simulink model "estimator_ekf_v04"  (Simulink 7.0)
settings: Solver=FixedStepDiscrete  StartTime=10  StopTime=20  FixedStep=1e-3  RelTol=1e-3
undefined symbols (not defined in the file): Ilf, Irf, P0, Q_in, R, ROBOT, ts, X0
libraries: simulink x6
settings Model: Creator=raje_ra  LastModifiedBy=raje_ra  ExtModeAutoUpdateStatusClock=off
settings DebuggingCC: SignalInfNanChecking=error  CheckMatrixSingularityMsg=warning

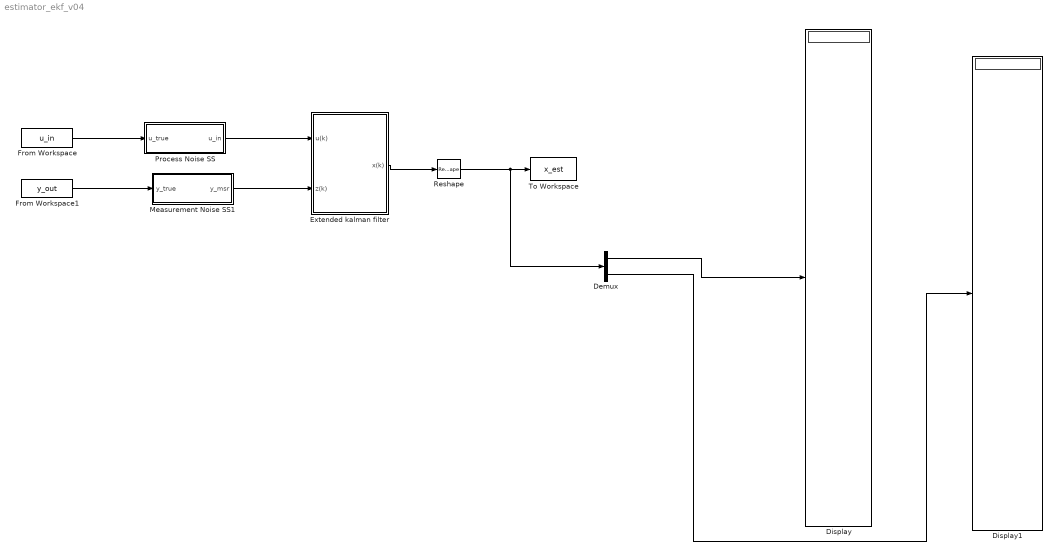
== system estimator_ekf_v04 ==
  Demux : Demux  Outputs=2
  Display : Display
  Display1 : Display
  Extended kalman filter : Subsystem
  From Workspace : FromWorkspace  VariableName=u_in  SampleTime=0
  From Workspace1 : FromWorkspace  VariableName=y_out  SampleTime=0
  Measurement Noise SS1 : Subsystem
  Process Noise SS : Subsystem
  Reshape : Reshape
  To Workspace : ToWorkspace  VariableName=x_est  SampleTime=-1  SaveFormat=Structure With Time
  wires:
  Extended kalman filter/1(x(k)) -> Reshape/1
  From Workspace1/1 -> Measurement Noise SS1/1(y_true)
  From Workspace/1 -> Process Noise SS/1(u_true)
  Reshape/1 -> To Workspace/1, Demux/1
  Measurement Noise SS1/1(y_msr) -> Extended kalman filter/2(z(k))
  Demux/1 -> Display/1
  Demux/2 -> Display1/1
  Process Noise SS/1(u_in) -> Extended kalman filter/1(u(k))

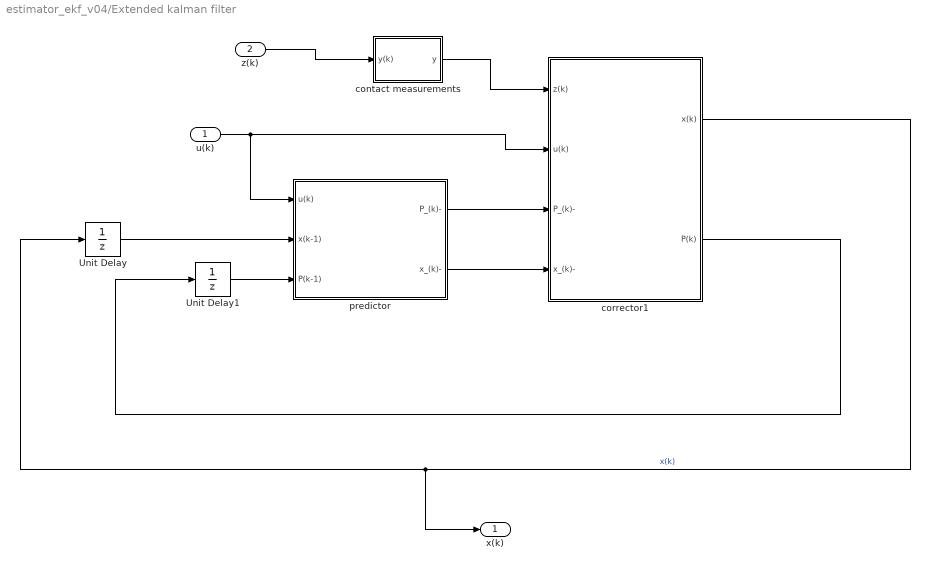
== system estimator_ekf_v04/Extended kalman filter ==
  u(k) : Inport  OutDataType=sfix(16)  OutScaling=2^0
  z(k) : Inport  Port=2  OutDataType=sfix(16)  OutScaling=2^0
  Unit Delay : UnitDelay  X0=X0  SampleTime=ts
  Unit Delay1 : UnitDelay  X0=P0  SampleTime=ts
  contact measurements : Subsystem
  corrector1 : Subsystem
  predictor : Subsystem
  x(k) : Outport  OutDataType=sfix(16)  OutScaling=2^0
  wires:
  u(k)/1 -> predictor/1(u(k)), corrector1/2(u(k))
  predictor/2(x_(k)-) -> corrector1/4(x_(k)-)
  Unit Delay/1 -> predictor/2(x(k-1))
  Unit Delay1/1 -> predictor/3(P(k-1))
  predictor/1(P_(k)-) -> corrector1/3(P_(k)-)
  corrector1/1(x(k)) -> Unit Delay/1, x(k)/1  "x(k)"
  z(k)/1 -> contact measurements/1(y(k))
  contact measurements/1(y) -> corrector1/1(z(k))
  corrector1/2(P(k)) -> Unit Delay1/1

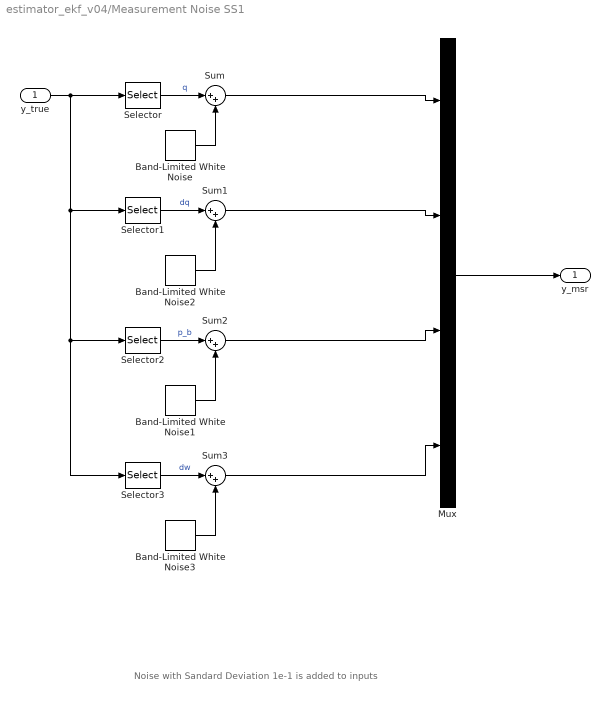
== system estimator_ekf_v04/Measurement Noise SS1 ==
  note: Noise with Sandard Deviation 1e-1 is added to inputs
  y_true : Inport  OutDataType=sfix(16)  OutScaling=2^0
  Band-Limited White Noise : simulink/Sources/Band-Limited White Noise  SystemSampleTime=-1  Cov=[1e-9]  Ts=ts  seed=[23341]
  Band-Limited White Noise1 : simulink/Sources/Band-Limited White Noise  SystemSampleTime=-1  Cov=[1e-5]  Ts=ts  seed=[23341]
  Band-Limited White Noise2 : simulink/Sources/Band-Limited White Noise  SystemSampleTime=-1  Cov=[1e-7]  Ts=ts  seed=[23341]
  Band-Limited White Noise3 : simulink/Sources/Band-Limited White Noise  SystemSampleTime=-1  Cov=[1e-7]  Ts=ts  seed=[23341]
  Mux : Mux
  Selector : Selector  InputPortWidth=m  IndexOptions=Index vector (dialog)  Indices=[1:25]  OutputSizes=1
  Selector1 : Selector  InputPortWidth=m  IndexOptions=Index vector (dialog)  Indices=[26:50]  OutputSizes=1
  Selector2 : Selector  InputPortWidth=m  IndexOptions=Index vector (dialog)  Indices=[51:53]  OutputSizes=1
  Selector3 : Selector  InputPortWidth=m  IndexOptions=Index vector (dialog)  Indices=[54:56]  OutputSizes=1
  Sum{,1..3} (4 alike) : Sum  Inputs=|++  OutDataType=sfix(16)  OutScaling=2^0
  y_msr : Outport
  wires:
  Mux/1 -> y_msr/1
  Sum3/1 -> Mux/4
  Sum2/1 -> Mux/3
  Sum1/1 -> Mux/2
  Sum/1 -> Mux/1
  Selector3/1 -> Sum3/1  "dw"
  Band-Limited White Noise3/1 -> Sum3/2
  Selector2/1 -> Sum2/1  "p_b"
  Band-Limited White Noise1/1 -> Sum2/2
  Band-Limited White Noise2/1 -> Sum1/2
  Selector1/1 -> Sum1/1  "dq"
  Selector/1 -> Sum/1  "q"
  y_true/1 -> Selector3/1, Selector2/1, Selector1/1, Selector/1
  Band-Limited White Noise/1 -> Sum/2

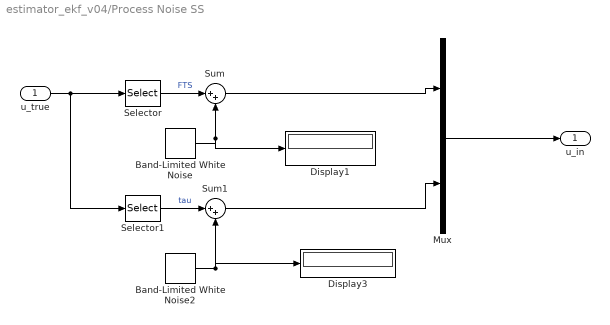
== system estimator_ekf_v04/Process Noise SS ==
  u_true : Inport  OutDataType=sfix(16)  OutScaling=2^0
  Band-Limited White Noise : simulink/Sources/Band-Limited White Noise  SystemSampleTime=-1  Cov=[1e-5]  Ts=ts  seed=[23341]
  Band-Limited White Noise2 : simulink/Sources/Band-Limited White Noise  SystemSampleTime=-1  Cov=[1e-6]  Ts=ts  seed=[23341]
  Display1 : Display
  Display3 : Display
  Mux : Mux  Inputs=2
  Selector : Selector  InputPortWidth=37  IndexOptions=Index vector (dialog)  Indices=[1:12]  OutputSizes=1
  Selector1 : Selector  InputPortWidth=37  IndexOptions=Index vector (dialog)  Indices=[13:37]  OutputSizes=1
  Sum : Sum  Inputs=|++  OutDataType=sfix(16)  OutScaling=2^0
  Sum1 : Sum  Inputs=|++  OutDataType=sfix(16)  OutScaling=2^0
  u_in : Outport
  wires:
  Mux/1 -> u_in/1
  Sum1/1 -> Mux/2
  Sum/1 -> Mux/1
  Band-Limited White Noise2/1 -> Display3/1, Sum1/2
  Selector1/1 -> Sum1/1  "tau"
  Selector/1 -> Sum/1  "FTS"
  u_true/1 -> Selector/1, Selector1/1
  Band-Limited White Noise/1 -> Display1/1, Sum/2

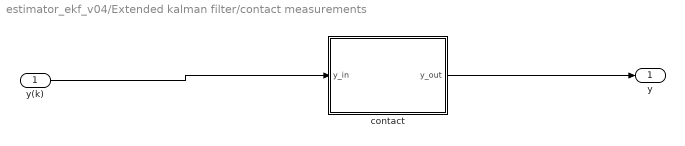
== system estimator_ekf_v04/Extended kalman filter/contact measurements ==
  y(k) : Inport
  contact : Subsystem  TreatAsAtomicUnit=on
  y : Outport
  wires:
  contact/1(y_out) -> y/1
  y(k)/1 -> contact/1(y_in)

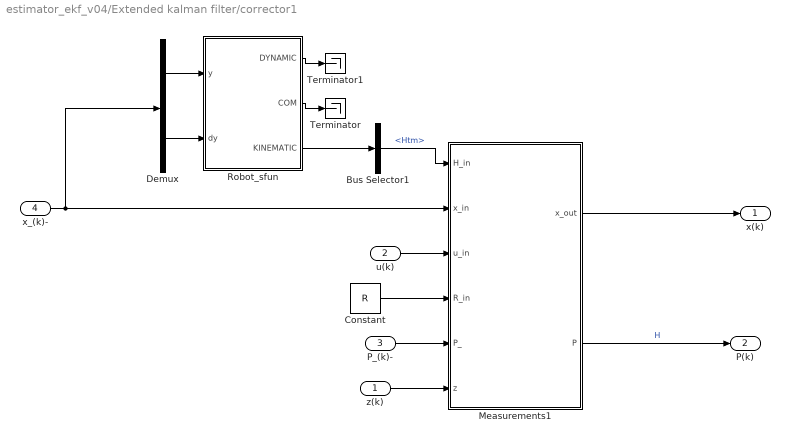
== system estimator_ekf_v04/Extended kalman filter/corrector1 ==
  z(k) : Inport  OutDataType=sfix(16)  OutScaling=2^0
  u(k) : Inport  Port=2  OutDataType=sfix(16)  OutScaling=2^0
  P_(k)- : Inport  Port=3  OutDataType=sfix(16)  OutScaling=2^0
  x_(k)- : Inport  Port=4  OutDataType=sfix(16)  OutScaling=2^0
  Bus Selector1 : BusSelector  OutputSignals=Htm
  Constant : Constant  Value=R  OutDataType=sfix(16)  OutScaling=2^0
  Demux : Demux  Outputs=2
  Measurements1 : Stateflow chart
  Robot_sfun : Subsystem
  Terminator : Terminator
  Terminator1 : Terminator
  x(k) : Outport  OutDataType=sfix(16)  OutScaling=2^0
  P(k) : Outport  Port=2  OutDataType=sfix(16)  OutScaling=2^0
  wires:
  Measurements1/2(P) -> P(k)/1  "H"
  z(k)/1 -> Measurements1/6(z)
  Constant/1 -> Measurements1/4(R_in)
  P_(k)-/1 -> Measurements1/5(P_)
  u(k)/1 -> Measurements1/3(u_in)
  Measurements1/1(x_out) -> x(k)/1
  x_(k)-/1 -> Measurements1/2(x_in), Demux/1
  Robot_sfun/2(COM) -> Terminator/1
  Demux/2 -> Robot_sfun/2(dy)
  Demux/1 -> Robot_sfun/1(y)
  Bus Selector1/1 -> Measurements1/1(H_in)  "<Htm>"
  Robot_sfun/3(KINEMATIC) -> Bus Selector1/1
  Robot_sfun/1(DYNAMIC) -> Terminator1/1

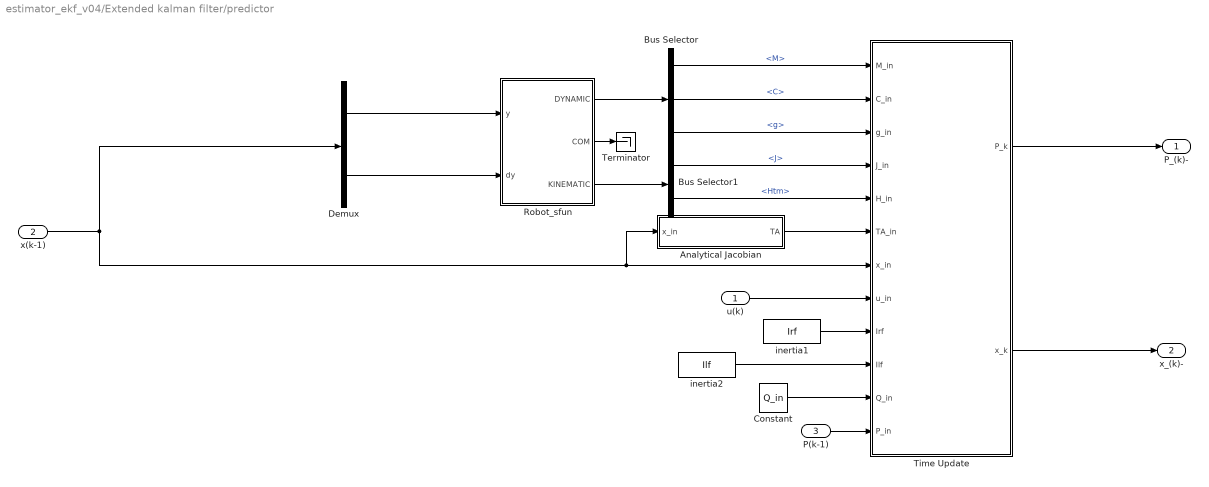
== system estimator_ekf_v04/Extended kalman filter/predictor ==
  u(k) : Inport  OutDataType=sfix(16)  OutScaling=2^0
  x(k-1) : Inport  Port=2  OutDataType=sfix(16)  OutScaling=2^0
  P(k-1) : Inport  Port=3  OutDataType=sfix(16)  OutScaling=2^0
  Analytical Jacobian : Stateflow chart
  Bus Selector : BusSelector  OutputSignals=M,C,g
  Bus Selector1 : BusSelector  OutputSignals=J,Htm
  Constant : Constant  Value=Q_in  VectorParams1D=off  OutDataType=sfix(16)  OutScaling=2^0
  Demux : Demux  Outputs=2
  Robot_sfun : Subsystem
  Terminator : Terminator
  Time Update : Stateflow chart
  inertia1 : Constant  Value=Irf  VectorParams1D=off  OutDataType=sfix(16)  OutScaling=2^0
  inertia2 : Constant  Value=Ilf  VectorParams1D=off  OutDataType=sfix(16)  OutScaling=2^0
  P_(k)- : Outport  OutDataType=sfix(16)  OutScaling=2^0
  x_(k)- : Outport  Port=2  OutDataType=sfix(16)  OutScaling=2^0
  wires:
  Time Update/1(P_k) -> P_(k)-/1
  Constant/1 -> Time Update/11(Q_in)
  P(k-1)/1 -> Time Update/12(P_in)
  Time Update/2(x_k) -> x_(k)-/1
  inertia2/1 -> Time Update/10(Ilf)
  inertia1/1 -> Time Update/9(Irf)
  u(k)/1 -> Time Update/8(u_in)
  Analytical Jacobian/1(TA) -> Time Update/6(TA_in)
  Robot_sfun/2(COM) -> Terminator/1
  Demux/2 -> Robot_sfun/2(dy)
  Demux/1 -> Robot_sfun/1(y)
  x(k-1)/1 -> Demux/1, Time Update/7(x_in), Analytical Jacobian/1(x_in)
  Bus Selector1/2 -> Time Update/5(H_in)  "<Htm>"
  Bus Selector1/1 -> Time Update/4(J_in)  "<J>"
  Robot_sfun/3(KINEMATIC) -> Bus Selector1/1
  Bus Selector/3 -> Time Update/3(g_in)  "<g>"
  Bus Selector/2 -> Time Update/2(C_in)  "<C>"
  Bus Selector/1 -> Time Update/1(M_in)  "<M>"
  Robot_sfun/1(DYNAMIC) -> Bus Selector/1

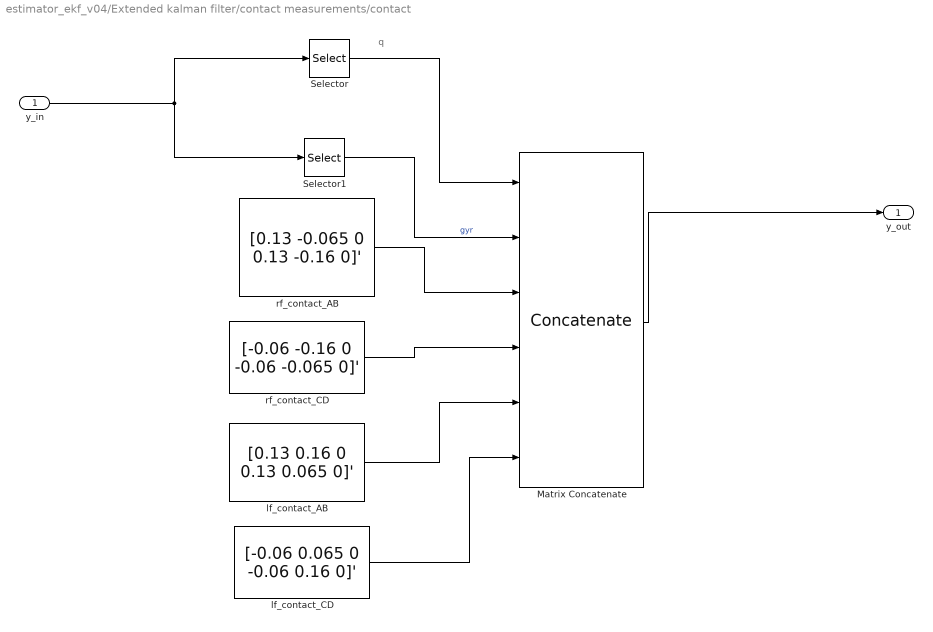
== system estimator_ekf_v04/Extended kalman filter/contact measurements/contact ==
  note: q
  y_in : Inport  OutDataType=sfix(16)  OutScaling=2^0
  Matrix Concatenate : Concatenate  NumInputs=6  Mode=Multidimensional array
  Selector : Selector  InputPortWidth=56  IndexOptions=Index vector (dialog)  Indices=1:25  OutputSizes=1
  Selector1 : Selector  InputPortWidth=56  IndexOptions=Index vector (dialog)  Indices=54:56  OutputSizes=1
  lf_contact_AB : Constant  Value="[0.13  0.16  0  0.13  0.065  0]'"  VectorParams1D=off  OutDataType=sfix(16)  OutScaling=2^0
  lf_contact_CD : Constant  Value="[-0.06  0.065  0  -0.06  0.16 0]'"  VectorParams1D=off  OutDataType=sfix(16)  OutScaling=2^0
  rf_contact_AB : Constant  Value="[0.13  -0.065  0   0.13  -0.16  0]'"  VectorParams1D=off  OutDataType=sfix(16)  OutScaling=2^0
  rf_contact_CD : Constant  Value="[-0.06  -0.16  0  -0.06  -0.065 0]'"  VectorParams1D=off  OutDataType=sfix(16)  OutScaling=2^0
  y_out : Outport  OutDataType=sfix(16)  OutScaling=2^0
  wires:
  lf_contact_CD/1 -> Matrix Concatenate/6
  lf_contact_AB/1 -> Matrix Concatenate/5
  rf_contact_CD/1 -> Matrix Concatenate/4
  rf_contact_AB/1 -> Matrix Concatenate/3
  Selector1/1 -> Matrix Concatenate/2  "gyr"
  Selector/1 -> Matrix Concatenate/1
  y_in/1 -> Selector1/1, Selector/1
  Matrix Concatenate/1 -> y_out/1

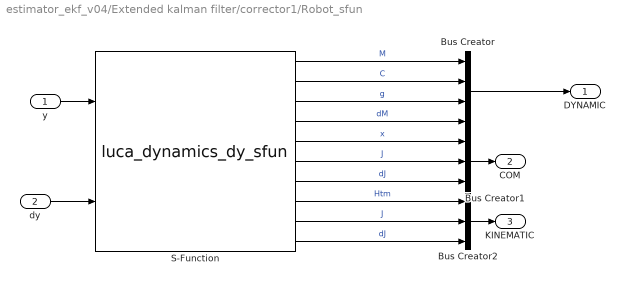
== system estimator_ekf_v04/Extended kalman filter/corrector1/Robot_sfun ==
  y : Inport
  dy : Inport  Port=2
  Bus Creator : BusCreator
  Bus Creator1 : BusCreator  Inputs=3
  Bus Creator2 : BusCreator  Inputs=3
  S-Function : S-Function  FunctionName=luca_dynamics_dy_sfun  Parameters=(size(ROBOT.csi,1)/6-1), size(ROBOT.csi,2), ROBOT.parent, ROBOT.tcp, ROBOT.g0, ROBOT.csi, ROBOT.com, ROBOT.Mass
  DYNAMIC : Outport
  COM : Outport  Port=2
  KINEMATIC : Outport  Port=3
  wires:
  Bus Creator2/1 -> KINEMATIC/1
  Bus Creator1/1 -> COM/1
  Bus Creator/1 -> DYNAMIC/1
  S-Function/10 -> Bus Creator2/3  "dJ"
  S-Function/9 -> Bus Creator2/2  "J"
  S-Function/8 -> Bus Creator2/1  "Htm"
  S-Function/7 -> Bus Creator1/3  "dJ"
  S-Function/6 -> Bus Creator1/2  "J"
  S-Function/5 -> Bus Creator1/1  "x"
  S-Function/4 -> Bus Creator/4  "dM"
  S-Function/3 -> Bus Creator/3  "g"
  S-Function/2 -> Bus Creator/2  "C"
  S-Function/1 -> Bus Creator/1  "M"
  dy/1 -> S-Function/2
  y/1 -> S-Function/1

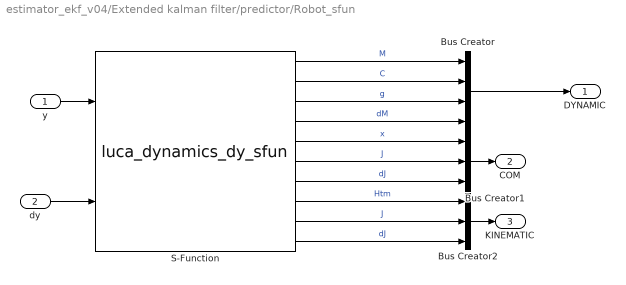
== system estimator_ekf_v04/Extended kalman filter/predictor/Robot_sfun ==
  y : Inport
  dy : Inport  Port=2
  Bus Creator : BusCreator
  Bus Creator1 : BusCreator  Inputs=3
  Bus Creator2 : BusCreator  Inputs=3
  S-Function : S-Function  FunctionName=luca_dynamics_dy_sfun  Parameters=(size(ROBOT.csi,1)/6-1), size(ROBOT.csi,2), ROBOT.parent, ROBOT.tcp, ROBOT.g0, ROBOT.csi, ROBOT.com, ROBOT.Mass
  DYNAMIC : Outport
  COM : Outport  Port=2
  KINEMATIC : Outport  Port=3
  wires:
  y/1 -> S-Function/1
  dy/1 -> S-Function/2
  S-Function/1 -> Bus Creator/1  "M"
  S-Function/2 -> Bus Creator/2  "C"
  S-Function/3 -> Bus Creator/3  "g"
  S-Function/4 -> Bus Creator/4  "dM"
  S-Function/5 -> Bus Creator1/1  "x"
  S-Function/6 -> Bus Creator1/2  "J"
  S-Function/7 -> Bus Creator1/3  "dJ"
  S-Function/8 -> Bus Creator2/1  "Htm"
  S-Function/9 -> Bus Creator2/2  "J"
  S-Function/10 -> Bus Creator2/3  "dJ"
  Bus Creator/1 -> DYNAMIC/1
  Bus Creator1/1 -> COM/1
  Bus Creator2/1 -> KINEMATIC/1

== matlab function Extended kalman filter/predictor/Analytical Jacobian ==
  data: TA output inherited; x_in input inherited
function TA = fcn(x_in)
% This block supports the Embedded MATLAB subset.
% See the help menu for details. 
% state - [ position ; velocity ]
% x_in  - [   1:31   ;   32:62  ]
ox = x_in(4);
oy = x_in(5);
% Transformation for Angular velocities to angular rates of floating base 
% on instantaneous frame of reference. x-y-z rotations.
%%{
T = [1      0           sin(oy);...
     0 cos(ox) -cos(oy)*sin(ox);...
     0 sin(ox)  cos(oy)*cos(ox)];


dTx = [0,         0,                0 ;...
       0,  -sin(ox),  -cos(oy)*cos(ox);...
       0,   cos(ox),  -cos(oy)*sin(ox)];
dTy = [0,         0,           cos(oy);...
       0,         0,   sin(oy)*sin(ox);...
       0,         0,  -sin(oy)*cos(ox)];
%%}

%{
T = [1      0   -sin(oy);...
     0  cos(ox)  cos(oy)*sin(ox);...
     0 -sin(ox)  cos(oy)*cos(ox)];
 
%T_A = [eye(3,6);zeros(3),T];

dTx = [0         0                0 ;
       0   -sin(ox)  cos(oy)*cos(ox);
       0   -cos(ox) -cos(oy)*sin(ox)];
dTy = [0       0        -cos(oy);
       0       0        -sin(oy)*sin(ox);
       0       0        -sin(oy)*cos(ox)];
%}

%TA = [ T_A; zeros(3*6,6); [zeros(3,6); [zeros(3) dTx]] ; [zeros(3,6); [zeros(3) dTy]]; zeros(57*6,6) ];

TA = [ T; dTx;dTy;zeros(3,3)];

== matlab function Extended kalman filter/predictor/Time Update ==
  data: P_k output inherited; M_in input inherited; x_k output inherited; C_in input inherited; g_in input inherited; J_in input inherited; H_in input inherited; TA_in input inherited; x_in input inherited; u_in input inherited; Irf input inherited; Ilf input inherited; Q_in input inherited; P_in input inherited
function [P_k,x_k]= fcn(M_in,C_in,g_in,J_in,H_in,TA_in,x_in,u_in,Irf,Ilf,Q_in,P_in)
% This block supports the Embedded MATLAB subset.
% See the help menu for details. 

dt = 1e-3;
dof = 31;
ind4 = -3:0;
ind6 = -5:0;

% Dynamic parameters
M = M_in(1:dof,:);
C = C_in(1:dof,:);
grav = g_in(1:dof);

invM = M \ eye(dof,dof);
% Kinematics
% tcp = 1 - Right Foot ; 2 - Left Foot ; 3 - Right Hand ; 4 - Left Hand ;
%       5 - Floating Base

Jrf = J_in(1*6+ind6,:);
Jlf = J_in(2*6+ind6,:);

Hrf = H_in(1*4+ind4,:);
Rrf = Hrf(1:3,1:3);
prf = Skew(Hrf(1:3,4));

Hlf = H_in(2*4+ind4,:);
Rlf = Hlf(1:3,1:3);
plf = Skew(Hlf(1:3,4));

Hfb = H_in(5*4+ind4,:);
Rfb = Hfb(1:3,1:3);

% state - [ position ; velocity ]
% x_in  - [   1:31   ;   32:62  ]
%q = x_in(1:dof);
dq = x_in(dof+(1:dof));

% inputs - [FTS_RF ; FTS _LF ; TRQ_JOINT]
% u_in   - [  1:6  ;   7:12  ;  13:37   ]
Frf = u_in(1*6+ind6,:);
Flf = u_in(2*6+ind6,:);
tau = [zeros(6,1); u_in(13:37)];

% Transformation for Angular velocities to angular rates of floating base 
% on instantaneous frame of reference. x-y-z rotations.
TA = TA_in(1:3,:);
invTA = TA \ eye(3,3);
% Transformation from body to spacial frame:
%Adfb = Adjoint(Hfb);
Adrf = Adjoint(Hrf);
Adlf = Adjoint(Hlf);

invAdrf = InvAdjoint(Hrf);
invAdlf = InvAdjoint(Hlf);

% Transformation for the velocites of floating base
vfb = dq(1:3);
wfb = dq(4:6);

dp = Rfb * vfb;
do = invTA * (Rfb*wfb);

vel = [dp; do; dq(7:31)];

%vel = [Vfb_s; dq(7:31)];%~~~~~~~ First Attempt

gacc = [ 0 0 -9.81 0 0 0]';
errrf = Irf * invAdrf * gacc ;
errlf = Ilf * invAdlf * gacc ;


% Computation of accelerations
acc = invM * (-C*dq - grav + tau + Jrf'*Adrf'*Frf + Jlf'*Adlf'*Flf - Jrf'*errrf - Jlf'*errlf);
x_dot = [vel;acc];   

% Computing second order derivative terms for base
% p - position of floating base o-orientation of floating base
x_k = x_in + dt*x_dot ;

% Computation the Jacobian of joint velocity function
dqdx = [zeros(25,37),eye(25)];                               %%%%%%%%%%%%%%%%

% Compute the Jacobian of acceleration terms(forward dynamics):
dpdx = zeros(3,2*dof);
dodx = zeros(3,2*dof);
dacc = zeros(dof,2*dof);
for i = 1:62
    dM   = M_in(i*dof+(1:dof),:);
    dC   = C_in(i*dof+(1:dof),:);
    dg   = g_in(i*dof+(1:dof));
    dJrf = J_in(i*30+(1*6+ind6),:);
    dJlf = J_in(i*30+(2*6+ind6),:);
    
    dHrf = H_in(i*20+(1*4+ind4),:);
    dRrf = dHrf(1:3,1:3);
    dprf = Skew(dHrf(1:3,4));
    dAdrf   = [ dRrf dprf*Rrf+prf*dRrf ; zeros(3) dRrf ];
    
    dHlf = H_in(i*20+(2*4+ind4),:); 
    dRlf = dHlf(1:3,1:3);
    dplf = Skew(dHlf(1:3,4));
    dAdlf   = [ dRlf dplf*Rlf+plf*dRlf ; zeros(3) dRlf ];
    
    dHfb  = H_in(i*20+(5*4+ind4),:); 
    dRfb  = dHfb( 1:3, 1:3);
 
    dpdx(:,i) = dRfb*vfb;
    dodx(:,i) = invTA * ( dRfb*wfb) ;

    if i > 3 && i < 6      
        dTA   = TA_in((i-3)*3+(1:3),:);
        dodx(:,i) = dodx(:,i) - invTA *(dTA*do );     % do = invTA * (Rfb*wfb);
    end 

      dacc(:,i)   = invM * (-dM*acc +(-dC*dq - dg + dJrf'*Adrf'*Frf + Jrf'*dAdrf'*Frf...
                                              + dJlf'*Adlf'*Flf + Jlf'*dAdlf'*Flf...
                                              - ( dJrf'*Irf* (invAdrf * gacc) + Jrf'*(-invAdrf *(dAdrf*(invAdrf * gacc))) ) ...
                                              - ( dJlf'*Ilf* (invAdlf * gacc) + Jlf'*(-invAdlf *(dAdlf*(invAdlf * gacc))) ) ));
    
    if i > dof
        if i <= dof+3
            dpdx(:,i) = dpdx(:,i) + Rfb(:,i-dof);         
        elseif i<= dof+6
            dodx(:,i) = dodx(:,i) + invTA * Rfb(:,i-(dof+3)); 
        end
        dacc(:,i) = dacc(:,i) + invM * (- C(:,i-31));

    end
end

dvel = [ dpdx ; dodx ; dqdx ];
A = eye(62) + dt * [dvel;dacc] ;

% Noise Correlation matrix
% tau_msr = tau_act + w_tau ==> tau_act = tau_msr -w_tau;
%dtau = invM*diag([zeros(6,1);ones(25,1)]);
W = [ zeros(dof,37); [-invM*Jrf'*Adrf' -invM*Jlf'*Adlf' -invM(:,7:end)] ];

P_k = A * P_in * A' + W * Q_in * W';

== matlab function Extended kalman filter/corrector1/Measurements1 ==
  data: x_out output inherited; H_in input inherited; x_in input inherited; u_in input inherited; P output inherited; R_in input inherited; P_ input inherited; z input inherited
function [x_out,P]= fcn(H_in,x_in,u_in,R_in,P_,z)
% This block supports the Embedded MATLAB subset.
% See the help menu for details. 

dof = 31;
ind4 = -3:0;
ind6 = -5:0;

% Kinematics
% tcp = 1 - Right Foot ; 2 - Left Foot ; 3 - Right Hand ; 4 - Left Hand ;
%       5 - Floating Base
Hrf = H_in(1*4+ind4,:);
Hlf = H_in(2*4+ind4,:);

% state - [ position ; velocity ]
% x_in  - [   1:31   ;   32:62  ]
q = x_in(1:dof);
dq = x_in(dof+(1:dof));
omega = dq(4:6);

% inputs - [FTS_RF ; FTS _LF ; TRQ_JOINT]
% u_in   - [  1:6  ;   7:12  ;  13:37   ]
Frf = u_in(1*6+ind6,:);
Flf = u_in(2*6+ind6,:);

gyro = omega;
 
%Internal sensors
jnt = q(7:31);

% Position of the contact points
% Contact Model:
%    x_ _        b---------c
%        |       |      .o |
%       y|       a---------d
%
% CD --> AB === Fx: 20 --> -20
% AB --> CD === Fx: -20 --> 20

contact_AB = [ 0.13 0.0475 0 1 0.13 -0.0475 0 1]';
contact_CD = [ -0.06 -0.0475 0 1 -0.06 0.0475 0 1]';

% zmp computation
zmprf_x = ( -Frf(5) -0.1189 * Frf(1) ) / Frf(3);
zmplf_x = ( -Flf(5) -0.1189 * Flf(1) ) / Flf(3);

zmp_x = (zmprf_x * Frf(3) + zmplf_x * Flf(3))/ (Frf(3)+Flf(3));

pa = contact_AB(1*4+ind4);
pb = contact_AB(2*4+ind4);
pc = contact_CD(1*4+ind4);
pd = contact_CD(2*4+ind4);

parf_s = Hrf * pa;
pbrf_s = Hrf * pb;
pcrf_s = Hrf * pc;
pdrf_s = Hrf * pd;

palf_s = Hlf * pa;
pblf_s = Hlf * pb;
pclf_s = Hlf * pc;
pdlf_s = Hlf * pd;

pcont = [ parf_s(1:3) ; pbrf_s(1:3) ; pcrf_s(1:3) ; pdrf_s(1:3) ;...
          palf_s(1:3) ; pblf_s(1:3) ; pclf_s(1:3) ; pdlf_s(1:3) ];

%measurement equation 
y = [ jnt ; gyro ; pcont];

% Compute the Jacobian of acceleration terms(forward dynamics):
dgyro = [ zeros(3,dof+3),eye(3,28) ];
dpcont = zeros(24,dof*2);

for i = 1:62
    dHrf = H_in(i*20+(1*4+ind4),:);
    dHlf = H_in(i*20+(2*4+ind4),:);

    dparf_s = dHrf*pa ; dpbrf_s = dHrf*pb ; dpcrf_s = dHrf*pc ; dpdrf_s = dHrf*pd ; 
    dpalf_s = dHlf*pa ; dpblf_s = dHlf*pb ; dpclf_s = dHlf*pc ; dpdlf_s = dHlf*pd;
    dpcont(:,i) =[ dparf_s(1:3) ; dpbrf_s(1:3) ; dpcrf_s(1:3) ; dpdrf_s(1:3) ;...
                   dpalf_s(1:3) ; dpblf_s(1:3) ; dpclf_s(1:3) ; dpdlf_s(1:3) ];
end

djnt =  [zeros(25,6),eye(25,25),zeros(25,31)]; 

if zmp_x < -0.05 
    % Pitching around back edge 
    C_uo = [ djnt ; dgyro ; dpcont([7:12 12+(7:12)],:)];
    R_uo = R_in(1:end-12,1:end-12);
    K_uo = P_*C_uo'/(C_uo*P_*C_uo'+R_uo);
    I = eye(size(P_));
    P = (I-K_uo*C_uo)*P_*(I-K_uo*C_uo)' + K_uo*R_uo*K_uo' ;
    x_out = x_in + K_uo *(z([1:28 28+[7:12 12+(7:12)]]) - y([1:28 28+[7:12 12+(7:12)]]));
elseif zmp_x> 0.12
    % Pitching around front edge 
    C_uo = [ djnt ; dgyro ; dpcont([1:6 12+(1:6)],:)];
    R_uo = R_in(1:end-12,1:end-12);
    K_uo = P_*C_uo'/(C_uo*P_*C_uo'+R_uo);
    I = eye(size(P_));
    P = (I-K_uo*C_uo)*P_*(I-K_uo*C_uo)' + K_uo*R_uo*K_uo' ;
    x_out = x_in + K_uo *(z([1:28 28+[1:6 12+(1:6)]]) - y([1:28 28+[1:6 12+(1:6)]]));
else
    %C_o = [ djnt ; dimu ; dgyro ; dpcont ; dvcont];
    C_o = [ djnt ; dgyro ; dpcont];
    R_o = R_in;
    K = P_*C_o'/(C_o*P_*C_o'+R_o);
    I = eye(size(P_));
    P = (I-K*C_o)*P_*(I-K*C_o)' + K*R_o*K' ;
    x_out = x_in + K *(z-y);
end
